simulink model "exercise4reabb"  (R2025b)
settings: Solver=VariableStepAuto  StartTime=0.0  StopTime=0.01  RelTol=1e-3
values from neighbouring files (symbols this model uses):
  cm = 23.4e-3    (= 0.0234)    [exer4creal.m]    (also in exercise4reab.m)
  D = 0.4191e-5    (= 4.191e-06)    [exer4creal.m]    (also in exercise4reab.m)
  J = 0.23e-6    (= 2.3e-07)    [exer4creal.m]    (also in exercise4reab.m)
  Kp = 0.05    [exer4creal.m]    (also in exercise4reab.m)
  L = 0.23e-3    (= 0.00023)    [exer4creal.m]    (also in exercise4reab.m)
  R = 2.4    [exer4creal.m]    (also in exercise4reab.m)
settings Model: Creator=Lenovo  LastModifiedBy=Lenovo

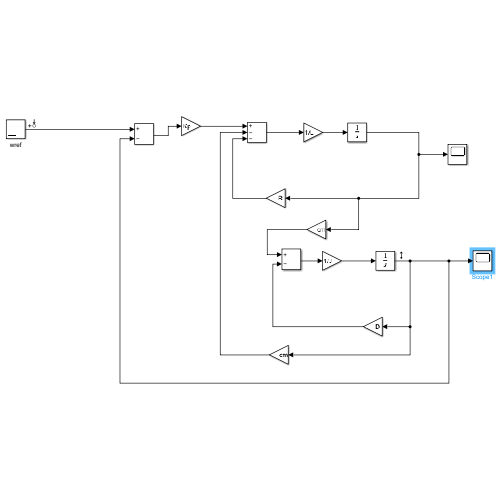
[thumbnail: Simulink's stored preview of the top-level diagram]
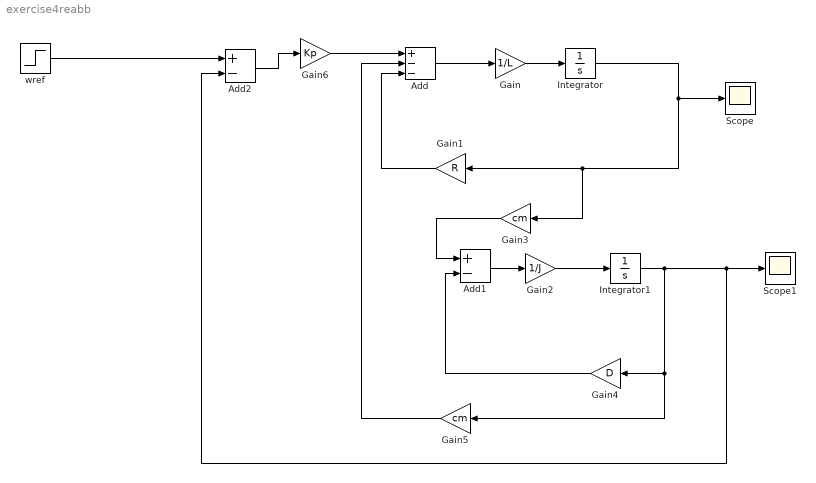
== system exercise4reabb ==
  Add : Sum  Inputs=+--
  Add1 : Sum  Inputs=+-
  Add2 : Sum  Inputs=+-
  Gain : Gain  Gain=1/L
  Gain1 : Gain  Gain=R
  Gain2 : Gain  Gain=1/J
  Gain3 : Gain  Gain=cm
  Gain4 : Gain  Gain=D
  Gain5 : Gain  Gain=cm
  Gain6 : Gain  Gain=Kp
  Integrator : Integrator
  Integrator1 : Integrator
  Scope : Scope
      settings: ActiveDisplayYMinimum=-1  ActiveDisplayYMaximum=1  DataLoggingVariableName=wx
  Scope1 : Scope
      settings: ActiveDisplayYMinimum=-1  ActiveDisplayYMaximum=1  DataLoggingVariableName=ex
  wref : Step  Time=0  After=300  SampleTime=0
  wires:
  Integrator/1 -> Gain3/1, Gain1/1, Scope/1
  Gain/1 -> Integrator/1
  Gain1/1 -> Add/3
  Gain3/1 -> Add1/1
  Add/1 -> Gain/1
  Gain4/1 -> Add1/2
  Gain2/1 -> Integrator1/1
  Add1/1 -> Gain2/1
  Gain5/1 -> Add/2
  Integrator1/1 -> Gain5/1, Gain4/1, Add2/2, Scope1/1
  wref/1 -> Add2/1
  Add2/1 -> Gain6/1
  Gain6/1 -> Add/1
